simulink model "controller_observer2"  (R2016b)
settings: Solver=ode45  StartTime=0.0  StopTime=10.0  RelTol=1e-3
values from neighbouring files (symbols this model uses):
  C = [1 0 0 0 0;0 0 1 0 0]    [cee_MACRO.m]
  D = [0 0 0 0 0]'    [cee_MACRO.m]
  T = 5    [cee_MACRO.m]
  x0 = degtorad(x0_graus)'    [cee_MACRO.m]
  x0c = deg2rad(x0c_graus)'    [cee_MACRO.m]
undefined symbols (not defined in the file or in its folder): A, Ac, B, Bc, Cc, Dc, perturbacao_alpha, perturbacao_beta
libraries: dspsrcs4 x3, powerlib_meascontrol x2
settings Model: Creator=jmgri  LastModifiedBy=jmgri
settings OptimizationCC: LifeSpan=inf
settings DebuggingCC: SFExecutionAtInitializationDiag=none
settings HardwareCC: ProdBitPerSizeT=32  ProdBitPerPtrDiffT=32  ProdWordSize=32  ProdHWDeviceType=Specified

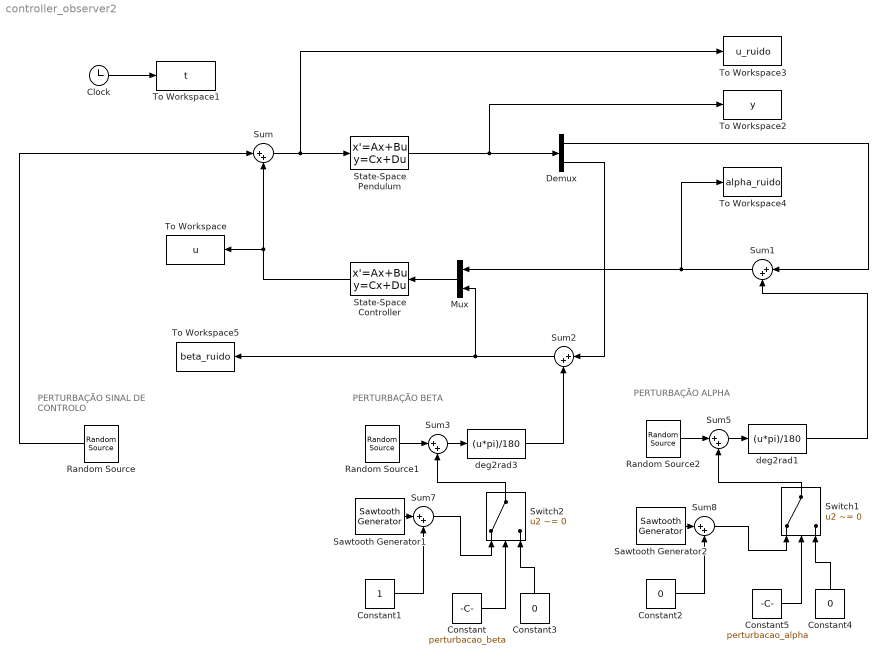
== system controller_observer2 ==
  note: PERTURBAÇÃO
      | SINAL DE CONTROLO
  note: PERTURBAÇÃO BETA
  note: PERTURBAÇÃO ALPHA
  Clock : Clock
  Constant : Constant  Value=perturbacao_beta
  Constant1 : Constant
  Constant2 : Constant  Value=0
  Constant3 : Constant  Value=0
  Constant4 : Constant  Value=0
  Constant5 : Constant  Value=perturbacao_alpha
  Demux : Demux  Outputs=2
  Mux : Mux  Inputs=2
  Random Source : dspsrcs4/Random Source  SrcType=Gaussian  NormMethod=Ziggurat  CltLength=12  MinVal=0  MaxVal=1  MeanVal=0  VarVal=1  RepMode=Not repeatable  rawSeed=1  IsInherit=off  SampMode=Continuous  SampTime=1  SampFrame=1  DataType=Double  OutComplex=Real  OutputFrames=off
  Random Source1 : dspsrcs4/Random Source  SrcType=Gaussian  NormMethod=Ziggurat  CltLength=12  MinVal=0  MaxVal=1  MeanVal=0  VarVal=1  RepMode=Not repeatable  rawSeed=1  IsInherit=off  SampMode=Continuous  SampTime=1  SampFrame=1  DataType=Double  OutComplex=Real  OutputFrames=off
  Random Source2 : dspsrcs4/Random Source  SrcType=Gaussian  NormMethod=Ziggurat  CltLength=12  MinVal=0  MaxVal=1  MeanVal=0  VarVal=1  RepMode=Not repeatable  rawSeed=1  IsInherit=off  SampMode=Continuous  SampTime=1  SampFrame=1  DataType=Double  OutComplex=Real  OutputFrames=off
  Sawtooth Generator1 : powerlib_meascontrol/Pulse & Signal Generators/Sawtooth Generator  Freq=0.5  Phase=180  Ts=T(length(T))
  Sawtooth Generator2 : powerlib_meascontrol/Pulse & Signal Generators/Sawtooth Generator  Freq=0.5  Phase=180  Ts=T(length(T))
  State-Space Controller : StateSpace  A=Ac  B=Bc  C=Cc  D=Dc  X0=x0c
  State-Space Pendulum : StateSpace  A=A  B=B  C=C  D=D  X0=x0
  Sum{,1..3,5,7..8} (7 alike) : Sum  Inputs=|++
  Switch1 : Switch  Criteria=u2 ~= 0
  Switch2 : Switch  Criteria=u2 ~= 0
  To Workspace : ToWorkspace  VariableName=u  SampleTime=-1
  To Workspace1 : ToWorkspace  VariableName=t  SampleTime=-1
  To Workspace2 : ToWorkspace  VariableName=y  SampleTime=-1
  To Workspace3 : ToWorkspace  VariableName=u_ruido  SampleTime=-1
  To Workspace4 : ToWorkspace  VariableName=alpha_ruido  SampleTime=-1
  To Workspace5 : ToWorkspace  VariableName=beta_ruido  SampleTime=-1
  deg2rad1 : Fcn  Expr=(u*pi)/180
  deg2rad3 : Fcn  Expr=(u*pi)/180
  wires:
  Clock/1 -> To Workspace1/1
  State-Space Pendulum/1 -> To Workspace2/1, Demux/1
  Sum/1 -> To Workspace3/1, State-Space Pendulum/1
  State-Space Controller/1 -> Sum/2, To Workspace/1
  Mux/1 -> State-Space Controller/1
  Demux/2 -> Sum2/1
  Sum1/1 -> To Workspace4/1, Mux/1
  Sum2/1 -> To Workspace5/1, Mux/2
  Demux/1 -> Sum1/1
  Random Source1/1 -> Sum3/1
  Sawtooth Generator1/1 -> Sum7/1
  Constant1/1 -> Sum7/2
  Sum3/1 -> deg2rad3/1
  deg2rad3/1 -> Sum2/2
  Random Source2/1 -> Sum5/1
  Sawtooth Generator2/1 -> Sum8/1
  Constant2/1 -> Sum8/2
  Sum5/1 -> deg2rad1/1
  deg2rad1/1 -> Sum1/2
  Random Source/1 -> Sum/1
  Switch2/1 -> Sum3/2
  Constant3/1 -> Switch2/3
  Constant/1 -> Switch2/2
  Sum7/1 -> Switch2/1
  Constant4/1 -> Switch1/3
  Constant5/1 -> Switch1/2
  Sum8/1 -> Switch1/1
  Switch1/1 -> Sum5/2
